simulink model "DT_DSM_CIFF_HIGH_PASS_MODEL_SECOND_ORDER_OSR_2048_FLICKER_NOISE"  (R2025b)
settings: Solver=VariableStepAuto  StartTime=0.0  StopTime=1  RelTol=1e-3
undefined symbols (not defined in the file): dspblkCoreblockFVToolHelper, gcbh
libraries: dspobslib x2, simulink_extras x1, cstblocks x1
settings Model: ModifiedByFormat=Team_33  Creator=Team_33  LastModifiedBy=Team_33

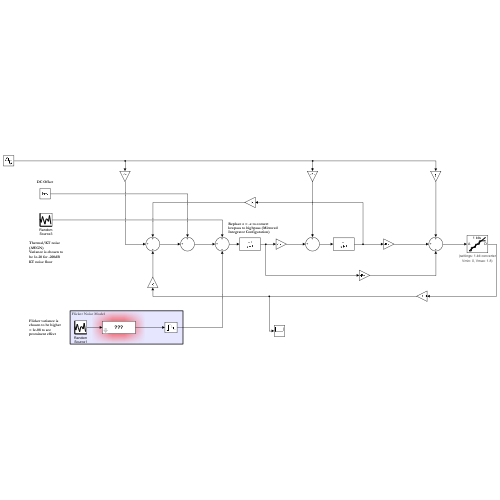
[thumbnail: Simulink's stored preview of the top-level diagram]
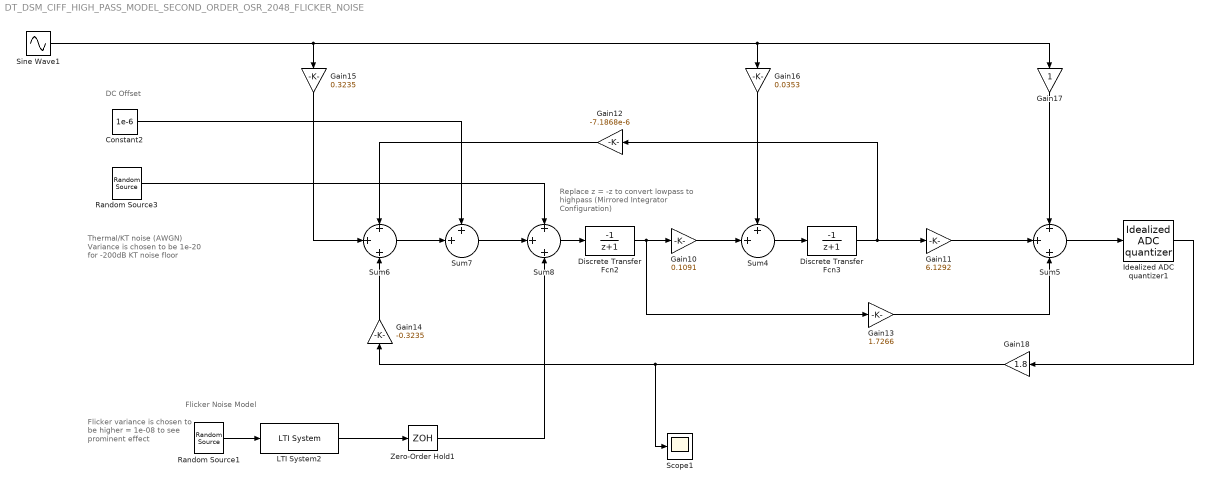
== system DT_DSM_CIFF_HIGH_PASS_MODEL_SECOND_ORDER_OSR_2048_FLICKER_NOISE ==
  note: Replace z = -z to convert lowpass to highpass (Mirrored Integrator Configuration)
  note: Thermal/KT noise
      | (AWGN)
      | Variance is chosen to
      | be 1e-20 for -200dB
      | KT noise floor
  note: Flicker Noise Model
  note: Flicker variance is
      | chosen to be higher
      | = 1e-08 to see
      | prominent effect
  note: DC Offset
  Constant2 : Constant  Value=1e-6
  Discrete Transfer Fcn2 : DiscreteTransferFcn  LoadFcn=dspblkCoreblockFVToolHelper(gcbh,'load');  Numerator=[-1]  Denominator=[1 1]
      settings: CopyFcn=dspblkCoreblockFVToolHelper(gcbh,'copy');  DeleteFcn=dspblkCoreblockFVToolHelper(gcbh,'close');  ModelCloseFcn=dspblkCoreblockFVToolHelper(gcbh,'close');  PreSaveFcn=dspblkCoreblockFVToolHelper(gcbh,'presave');  PostSaveFcn=dspblkCoreblockFVToolHelper(gcbh,'postsave');  CloseFcn=dspblkCoreblockFVToolHelper(gcbh,'close');
  Discrete Transfer Fcn3 : DiscreteTransferFcn  LoadFcn=dspblkCoreblockFVToolHelper(gcbh,'load');  Numerator=[-1]  Denominator=[1 1]
      settings: CopyFcn=dspblkCoreblockFVToolHelper(gcbh,'copy');  DeleteFcn=dspblkCoreblockFVToolHelper(gcbh,'close');  ModelCloseFcn=dspblkCoreblockFVToolHelper(gcbh,'close');  PreSaveFcn=dspblkCoreblockFVToolHelper(gcbh,'presave');  PostSaveFcn=dspblkCoreblockFVToolHelper(gcbh,'postsave');  CloseFcn=dspblkCoreblockFVToolHelper(gcbh,'close');
  Gain10 : Gain  Gain=0.1091
  Gain11 : Gain  Gain=6.1292
  Gain12 : Gain  Gain=-7.1868e-6
  Gain13 : Gain  Gain=1.7266
  Gain14 : Gain  Gain=-0.3235
  Gain15 : Gain  Gain=0.3235
  Gain16 : Gain  Gain=0.0353
  Gain17 : Gain
  Gain18 : Gain  Gain=1.8
  Idealized ADC quantizer1 : simulink_extras/Additional Discrete/Idealized ADC quantizer  NumberOfConverterBits=1  Vmin=0  Vmax=1.8  OutputDataType=int16  OutputNegativeValues=off
  LTI System2 : cstblocks/LTI System  sys=ff_ss  IC=[]  PadeOrder=0
  Random Source1 : dspobslib/Random Source  SrcType=Gaussian  NormMethod=Ziggurat  CltLength=12  MinVal=0  MaxVal=1  MeanVal=0  VarVal=1e-8  RepMode=Not repeatable  rawSeed=1  IsInherit=off  SampMode=Discrete  SampTime=1/(2000*2048)  SampFrame=1  DataType=Double  OutComplex=Real  OutputFrames=off
  Random Source3 : dspobslib/Random Source  SrcType=Gaussian  NormMethod=Ziggurat  CltLength=12  MinVal=0  MaxVal=1  MeanVal=0  VarVal=1e-20  RepMode=Not repeatable  rawSeed=1  IsInherit=off  SampMode=Discrete  SampTime=1/(2000*2048)  SampFrame=1  DataType=Double  OutComplex=Real  OutputFrames=off
  Scope1 : Scope
      settings: ActiveDisplayYMinimum=1.03994  ActiveDisplayYMaximum=1.04051  DataLoggingVariableName=output_data  DataLoggingSaveFormat=Array
  Sine Wave1 : Sin  Amplitude=0.3  Bias=0.9  Frequency=(2000*2048)*(2*pi*127)/(32768*32) + 2*pi*(2048*2000)/2  SampleTime=1/(2000*2048)
  Sum4 : Sum  Inputs=++|
  Sum5 : Sum  Inputs=+|+|+
  Sum6 : Sum  Inputs=+|+|+
  Sum7 : Sum  Inputs=++|
  Sum8 : Sum  Inputs=+|+|+
  Zero-Order Hold1 : ZeroOrderHold  SampleTime=1/(2000*2048)
  wires:
  LTI System2/1 -> Zero-Order Hold1/1
  Sum8/1 -> Discrete Transfer Fcn2/1
  Discrete Transfer Fcn3/1 -> Gain12/1, Gain11/1
  Zero-Order Hold1/1 -> Sum8/3
  Random Source1/1 -> LTI System2/1
  Constant2/1 -> Sum7/1
  Sum6/1 -> Sum7/2
  Gain17/1 -> Sum5/1
  Gain11/1 -> Sum5/2
  Gain14/1 -> Sum6/3
  Random Source3/1 -> Sum8/1
  Gain16/1 -> Sum4/1
  Sum7/1 -> Sum8/2
  Gain10/1 -> Sum4/2
  Sum5/1 -> Idealized ADC quantizer1/1
  Discrete Transfer Fcn2/1 -> Gain10/1, Gain13/1
  Gain18/1 -> Scope1/1, Gain14/1
  Gain15/1 -> Sum6/2
  Sine Wave1/1 -> Gain17/1, Gain16/1, Gain15/1
  Idealized ADC quantizer1/1 -> Gain18/1
  Gain12/1 -> Sum6/1
  Gain13/1 -> Sum5/3
  Sum4/1 -> Discrete Transfer Fcn3/1
